simulink library "ESTS_UOD_AgrVSideSlipReDifLatRef"  (R2022a)
settings: Solver=VariableStepAuto  StartTime=0.0  StopTime=10.0  RelTol=1e-3
undefined symbols (not defined in the file): ESTS_UOD_p_AgrVSideSlipReDifLowLim_radps, ESTS_UOD_p_AgrVSideSlipReLowLim_radps
settings Model: Creator=blatak  LastModifiedBy=blatak

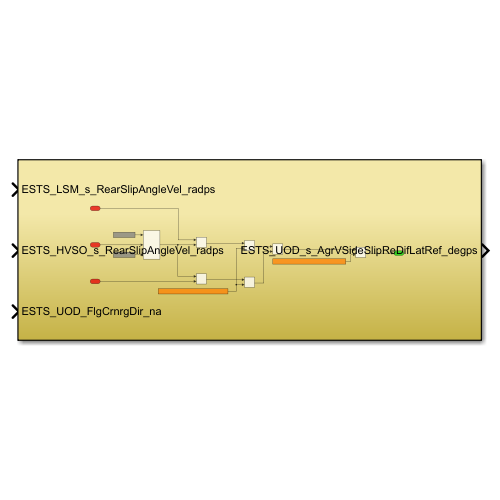
[thumbnail: Simulink's stored preview of the top-level diagram]
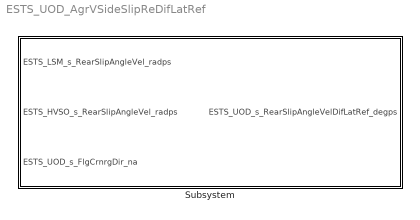
== system ESTS_UOD_AgrVSideSlipReDifLatRef ==
  Subsystem : Subsystem

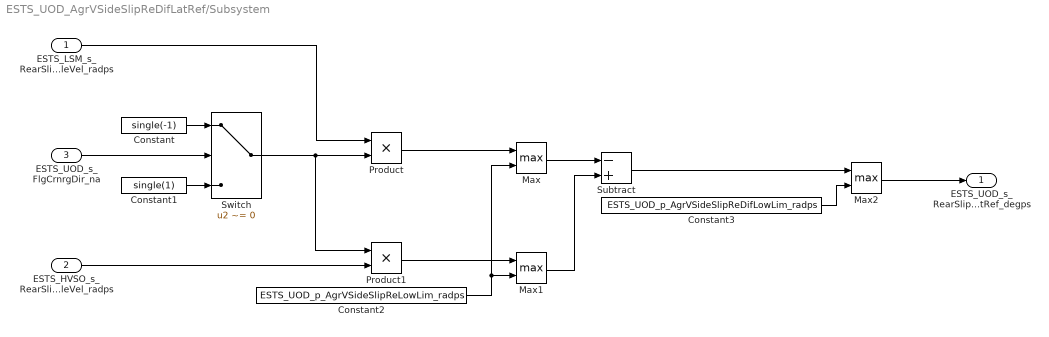
== system ESTS_UOD_AgrVSideSlipReDifLatRef/Subsystem ==
  ESTS_LSM_s_RearSlipAngleVel_radps : Inport
  ESTS_HVSO_s_RearSlipAngleVel_radps : Inport  Port=2
  ESTS_UOD_s_FlgCrnrgDir_na : Inport  Port=3
  Constant : Constant  Value=single(-1)
  Constant1 : Constant  Value=single(1)
  Constant2 : Constant  Value=ESTS_UOD_p_AgrVSideSlipReLowLim_radps
  Constant3 : Constant  Value=ESTS_UOD_p_AgrVSideSlipReDifLowLim_radps
  Max : MinMax  Function=max  Inputs=2
  Max1 : MinMax  Function=max  Inputs=2
  Max2 : MinMax  Function=max  Inputs=2
  Product : Product
  Product1 : Product
  Subtract : Sum  Inputs=-+
  Switch : Switch  Criteria=u2 ~= 0  SaturateOnIntegerOverflow=off  InputSameDT=off
  ESTS_UOD_s_RearSlipAngleVelDifLatRef_degps : Outport
  wires:
  ESTS_UOD_s_FlgCrnrgDir_na/1 -> Switch/2
  Switch/1 -> Product1/1, Product/2
  Constant1/1 -> Switch/3
  Constant/1 -> Switch/1
  Product/1 -> Max/1
  ESTS_LSM_s_RearSlipAngleVel_radps/1 -> Product/1
  Constant3/1 -> Max2/2
  Constant2/1 -> Max/2, Max1/2
  ESTS_HVSO_s_RearSlipAngleVel_radps/1 -> Product1/2
  Max2/1 -> ESTS_UOD_s_RearSlipAngleVelDifLatRef_degps/1
  Product1/1 -> Max1/1
  Subtract/1 -> Max2/1
  Max1/1 -> Subtract/2
  Max/1 -> Subtract/1
